simulink model "sim_linear_control3"  (R2018a)
settings: Solver=ode3  StartTime=0.0  StopTime=5  FixedStep=0.001  RelTol=1e-3
values from neighbouring files (symbols this model uses):
  C = [1 0 ... (first row only)    [lin_control.m]    (also in lin_control3.m = [0 1])
  CA = C*A    [lin_control.m]    (also in lin_control3.m)
  fc = 0.5    [lin_control.m]    (also in lin_control3.m)
  invCB = pinv(C*B)    [lin_control.m]    (also in lin_control3.m)
  Kb = 4    [lin_control.m]    (also in lin_control3.m)
settings Model: Creator=E183308  LastModifiedBy=E183308

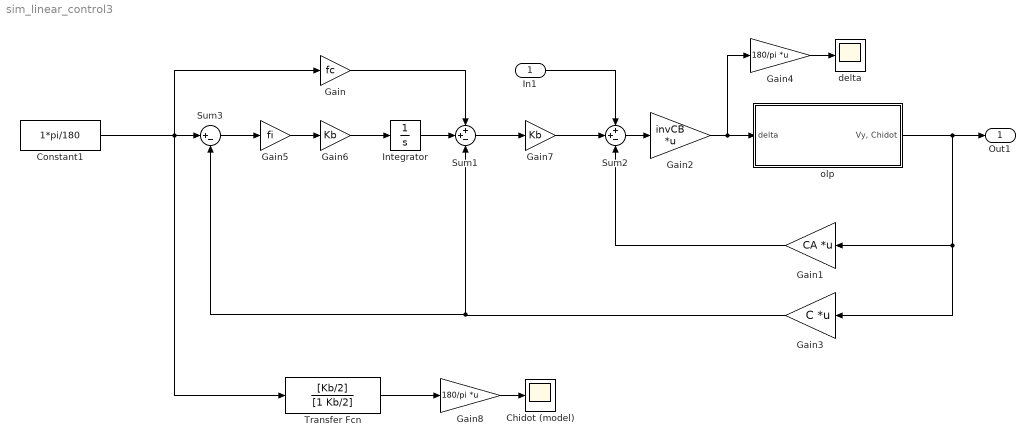
== system sim_linear_control3 ==
  In1 : Inport
  Chidot (model) : Scope
  Constant1 : Constant  Value=1*pi/180
  Gain : Gain  Gain=fc
  Gain1 : Gain  Gain=CA  Multiplication=Matrix(K*u)
  Gain2 : Gain  Gain=invCB  Multiplication=Matrix(K*u)
  Gain3 : Gain  Gain=C  Multiplication=Matrix(K*u)
  Gain4 : Gain  Gain=180/pi  Multiplication=Matrix(K*u)
  Gain5 : Gain  Gain=fi
  Gain6 : Gain  Gain=Kb
  Gain7 : Gain  Gain=Kb
  Gain8 : Gain  Gain=180/pi  Multiplication=Matrix(K*u)
  Integrator : Integrator
  Sum1 : Sum  Inputs=++-
  Sum2 : Sum  Inputs=++-
  Sum3 : Sum  Inputs=|+-
  Transfer Fcn : TransferFcn  Numerator=[Kb/2]  Denominator=[1 Kb/2]
  delta : Scope
  olp : Subsystem
  Out1 : Outport
  wires:
  Sum2/1 -> Gain2/1
  Gain2/1 -> Gain4/1, olp/1(delta)
  olp/1("Vy, Chidot") -> Gain3/1, Gain1/1, Out1/1
  Gain4/1 -> delta/1
  Gain7/1 -> Sum2/2
  Gain1/1 -> Sum2/3
  In1/1 -> Sum2/1
  Gain/1 -> Sum1/1
  Gain5/1 -> Gain6/1
  Integrator/1 -> Sum1/2
  Gain6/1 -> Integrator/1
  Sum3/1 -> Gain5/1
  Constant1/1 -> Transfer Fcn/1, Gain/1, Sum3/1
  Sum1/1 -> Gain7/1
  Gain3/1 -> Sum3/2, Sum1/3
  Gain8/1 -> Chidot (model)/1
  Transfer Fcn/1 -> Gain8/1

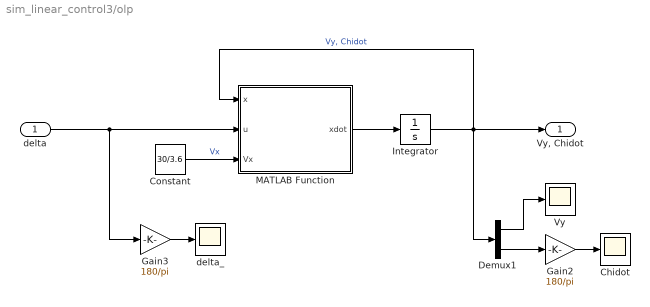
== system sim_linear_control3/olp ==
  delta : Inport
  Chidot : Scope
  Constant : Constant  Value=30/3.6
  Demux1 : Demux  Outputs=2
  Gain2 : Gain  Gain=180/pi
  Gain3 : Gain  Gain=180/pi
  Integrator : Integrator  InitialCondition=[0;0]
  MATLAB Function : MATLAB Function  TreatAsAtomicUnit=on
  Vy : Scope
  delta_ : Scope
  "Vy, Chidot" : Outport
  wires:
  Gain2/1 -> Chidot/1
  Demux1/2 -> Gain2/1
  Integrator/1 -> MATLAB Function/1(x), "Vy, Chidot"/1, Demux1/1  "Vy, Chidot"
  Gain3/1 -> delta_/1
  delta/1 -> Gain3/1, MATLAB Function/2(u)
  Constant/1 -> MATLAB Function/3(Vx)  "Vx"
  MATLAB Function/1(xdot) -> Integrator/1
  Demux1/1 -> Vy/1

== matlab function sim_linear_control3/olp/MATLAB Function ==
  data: x input; u input; xdot output; Vx input
function xdot = dynamic_lin(x,u,Vx)

% sports sedan

m = 1724; % kg
Iz = 3400; % kg/m^2
a = 1.35; % m
b = 1.15; % m
Cf = 12*1e4; % N/rad
Cr = 175*1e3; % N/rad
mu = 0.5225;

% x = [vy Chidot], u = delta

A = [-(Cf+Cr)/m  -(a*Cf-b*Cr)/(m*Vx)-Vx; 
    -(a*Cf-b*Cr)/(Iz*Vx) -(a^2*Cf-b^2*Cr)/(Iz*Vx)];

B = [Cf/m; a*Cf/Iz];

xdot = A*x + B*u;
